simulink model "frecuencia_intermedia"  (R2021a)
settings: Solver=VariableStepAuto  StartTime=0.0  StopTime=10.0  RelTol=1e-3
libraries: commfilt2 x2
settings Model: Creator=Bremdows  LastModifiedBy=Bremdows

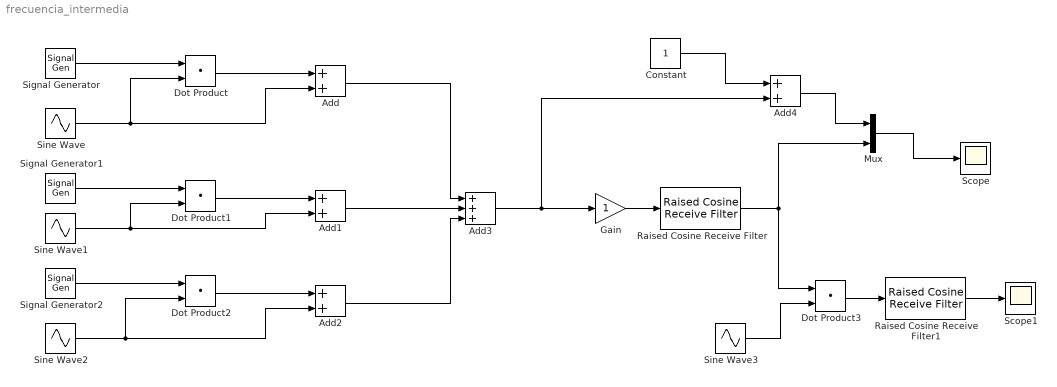
== system frecuencia_intermedia ==
  Add{,1..2,4} (4 alike) : Sum
  Add3 : Sum  Inputs=+++
  Constant : Constant
  Dot Product{,1..3} (4 alike) : DotProduct  InputSameDT=on  OutDataTypeStr=Inherit: Inherit via internal rule
  Gain : Gain
  Mux : Mux  Inputs=2
  Raised Cosine Receive Filter : commfilt2/Raised Cosine Receive Filter  filtType=Square root  R=0.2  filtSpan=10  N=8  downFactor=1  downOffset=0  filterGain=1  InputProcessing=Columns as channels (frame based)  RateOptions=Enforce single-rate processing  framing=Mute  checkCoeff=off  variableName=rcRxFilt  currentFiltSpan=10  D=5  inputOffset=0  sampMode=Mute  saveAsFlag=0  rateMode=Downsampling  checkGain=Normalized  launchFVT=on  roundingMode=Floor  overflowMode=off  coeffDataTypeStr=Inherit: Same word length as input  coeffMin=[]  coeffMax=[]  coeffLastDataTypeStr=Inherit: Same word length as input  accumDataTypeStr=Inherit: Same as product output  accumLastDataTypeStr=Inherit: Same as product output  outputDataTypeStr=Inherit: Same as accumulator  outputMin=[]  outputMax=[]  outputLastDataTypeStr=Inherit: Same as accumulator
  Raised Cosine Receive Filter1 : commfilt2/Raised Cosine Receive Filter  filtType=Square root  R=0.2  filtSpan=10  N=8  downFactor=1  downOffset=0  filterGain=1  InputProcessing=Columns as channels (frame based)  RateOptions=Enforce single-rate processing  framing=Mute  checkCoeff=off  variableName=rcRxFilt1  currentFiltSpan=10  D=5  inputOffset=0  sampMode=Mute  saveAsFlag=0  rateMode=Downsampling  checkGain=Normalized  launchFVT=on  roundingMode=Floor  overflowMode=off  coeffDataTypeStr=Inherit: Same word length as input  coeffMin=[]  coeffMax=[]  coeffLastDataTypeStr=Inherit: Same word length as input  accumDataTypeStr=Inherit: Same as product output  accumLastDataTypeStr=Inherit: Same as product output  outputDataTypeStr=Inherit: Same as accumulator  outputMin=[]  outputMax=[]  outputLastDataTypeStr=Inherit: Same as accumulator
  Scope : Scope
  Scope1 : Scope
  Signal Generator : SignalGenerator  Frequency=4e3  Units=rad/sec
  Signal Generator1 : SignalGenerator  Frequency=4e3  Units=rad/sec
  Signal Generator2 : SignalGenerator  Frequency=4e3  Units=rad/sec
  Sine Wave : Sin  Frequency=10e3  SampleTime=0
  Sine Wave1 : Sin  Frequency=20e3  SampleTime=0
  Sine Wave2 : Sin  Frequency=30e3  SampleTime=0
  Sine Wave3 : Sin  SampleTime=0
  wires:
  Sine Wave/1 -> Add/2, Dot Product/2
  Sine Wave1/1 -> Add1/2, Dot Product1/2
  Sine Wave2/1 -> Add2/2, Dot Product2/2
  Constant/1 -> Add4/1
  Add3/1 -> Add4/2, Gain/1
  Add/1 -> Add3/1
  Add1/1 -> Add3/2
  Add2/1 -> Add3/3
  Dot Product1/1 -> Add1/1
  Dot Product/1 -> Add/1
  Dot Product2/1 -> Add2/1
  Signal Generator/1 -> Dot Product/1
  Signal Generator1/1 -> Dot Product1/1
  Signal Generator2/1 -> Dot Product2/1
  Add4/1 -> Mux/1
  Mux/1 -> Scope/1
  Sine Wave3/1 -> Dot Product3/2
  Gain/1 -> Raised Cosine Receive Filter/1
  Raised Cosine Receive Filter/1 -> Dot Product3/1, Mux/2
  Raised Cosine Receive Filter1/1 -> Scope1/1
  Dot Product3/1 -> Raised Cosine Receive Filter1/1
